simulink model "P2"  (R2014a)
settings: Solver=ode23t  StartTime=0.0  StopTime=0.1  RelTol=1e-3
undefined symbols (not defined in the file): Ts
libraries: powerlib x17, powerlib_extras x5, fl_lib x4, elec_lib x4, nesl_utility x2
settings Model: Creator=HP  LastModifiedBy=HP

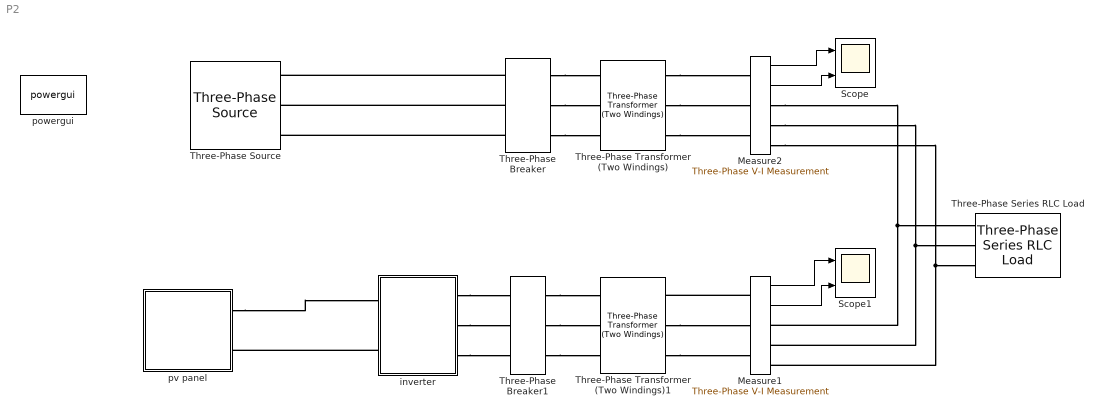
== system P2 ==
  Measure1 : powerlib/Measurements/Three-Phase V-I Measurement  VoltageMeasurement=phase-to-ground  SetLabelV=off  LabelV=V1  Vpu=off  VpuLL=off  CurrentMeasurement=yes  SetLabelI=off  LabelI=I1  Ipu=off  Pbase=1e3  Vbase=380  OutputType=Magnitude  PhasorSimulation=off  PSBequivalent=0
  Measure2 : powerlib/Measurements/Three-Phase V-I Measurement  VoltageMeasurement=phase-to-ground  SetLabelV=off  LabelV=V1  Vpu=off  VpuLL=off  CurrentMeasurement=yes  SetLabelI=off  LabelI=I1  Ipu=off  Pbase=1e3  Vbase=380  OutputType=Magnitude  PhasorSimulation=off  PSBequivalent=0
  Scope : Scope  NumInputPorts=2
      settings: YMin=-5000~-35  YMax=8000~55  SaveName=ScopeData4
  Scope1 : Scope  NumInputPorts=2
      settings: YMin=-2.25~-0.05  YMax=2.75~0.04  SaveName=ScopeData5
  Three-Phase Series RLC Load : powerlib/Elements/Three-Phase Series RLC Load  LConnTagsString=A|B|C  Configuration=Y (grounded)  NominalVoltage=380  NominalFrequency=50  ActivePower=1e3  InductivePower=0  CapacitivePower=0  Measurements=None  LoadType=constant Z
  Three-Phase Transformer (Two Windings) : powerlib/Elements/Three-Phase Transformer (Two Windings)  Winding1Connection=Yg  UNITS=pu  NominalPower=[ 250e6 , 60 ]  Winding1=[ 735e3 , 0.002 , 0.08 ]  Winding2Connection=Yg  Winding2=[ 315e3 , 0.002 , 0.08 ]  SetSaturation=off  Rm=500  Lm=500  Saturation=[ 0,0 ; 0.0024,1.2 ; 1.0,1.52 ]  Hysteresis=off  DataFile='hysteresis'  SetInitialFlux=off  InitialFluxes=[ 0.8 , -0.8 , 0.7 ]  Measurements=None  MoreParameters=off  BreakLoop=off  DataType=off  TransfoNumber=1
  Three-Phase Transformer (Two Windings)1 : powerlib/Elements/Three-Phase Transformer (Two Windings)  Winding1Connection=Yg  UNITS=pu  NominalPower=[ 250e6 , 60 ]  Winding1=[ 735e3 , 0.002 , 0.08 ]  Winding2Connection=Yg  Winding2=[ 315e3 , 0.002 , 0.08 ]  SetSaturation=off  Rm=500  Lm=500  Saturation=[ 0,0 ; 0.0024,1.2 ; 1.0,1.52 ]  Hysteresis=off  DataFile='hysteresis'  SetInitialFlux=off  InitialFluxes=[ 0.8 , -0.8 , 0.7 ]  Measurements=None  MoreParameters=off  BreakLoop=off  DataType=off  TransfoNumber=1
  Three-Phase Breaker : powerlib/Elements/Three-Phase Breaker  InitialState=open  SwitchA=on  SwitchB=on  SwitchC=on  SwitchTimes="[4/60  10/60]"  External=off  BreakerResistance=0.001  SnubberResistance=1e6  SnubberCapacitance=inf  Measurements=None
  Three-Phase Breaker1 : powerlib/Elements/Three-Phase Breaker  InitialState=closed  SwitchA=on  SwitchB=on  SwitchC=on  SwitchTimes="[4/60  10/60]"  External=off  BreakerResistance=0.001  SnubberResistance=1e6  SnubberCapacitance=inf  Measurements=None
  Three-Phase Source : powerlib/Electrical Sources/Three-Phase Source  Voltage=25e3  PhaseAngle=0  Frequency=60  InternalConnection=Yg  SpecifyImpedance=on  Resistance=0.8929  Inductance=16.58e-3  ShortCircuitLevel=100e6  BaseVoltage=25e3  XRratio=7  BusType=swing  Pref=0  Qref=0  Qmin=-inf  Qmax=inf
  inverter : Subsystem
  powergui : powerlib/powergui  Priority=1  SimulationMode=Continuous  SolverType=Tustin  SampleTime=50e-6  frequency=60  SPID=off  DisableSnubberDevices=off  DisableRonSwitches=off  DisableVfSwitches=off  SwTol=0  Interpol=off  DisplayEquations=off  Ts=0  methode=off  frequencyindice=0  Pbase=100e6  ErrMax=1e-4  Iterations=50  UnitsV=kV  UnitsW=MW  FunctionMessages=off  echomessages=off  HookPort=off  EnableUseOfTLC=off  x0status=blocks  RestoreLinks=warning  ResistiveCurrentMeasurement=off  Frange=[0:2:500]  Ylog=off  Xlog=on  ShowGrid=off  save=off  variable=ZData  structure=0  ZoomFFT=off  StartTime=0.0  cycles=1  DisplayStyle=1  fundamental=60  FreqAxis=off  MaxFrequency=1000  frequencyindicesteady=1  RmsSteady=1  display=off
  pv panel : Subsystem
  wires:
  Measure2/1 -> Scope/1
  Measure2/2 -> Scope/2
  Measure1/2 -> Scope1/2
  Measure1/1 -> Scope1/1
  connections:
  Measure2/RConn3 -- Measure1/RConn3 -- Three-Phase Series RLC Load/LConn3
  Measure2/RConn2 -- Measure1/RConn2 -- Three-Phase Series RLC Load/LConn2
  Measure2/RConn1 -- Measure1/RConn1 -- Three-Phase Series RLC Load/LConn1
  Three-Phase Breaker/LConn3 -- Three-Phase Source/RConn3
  Three-Phase Breaker/LConn2 -- Three-Phase Source/RConn2
  Three-Phase Breaker/LConn1 -- Three-Phase Source/RConn1
  inverter/RConn1 -- Three-Phase Breaker1/LConn1
  inverter/RConn2 -- Three-Phase Breaker1/LConn2
  inverter/RConn3 -- Three-Phase Breaker1/LConn3
  Three-Phase Breaker1/RConn1 -- Three-Phase Transformer (Two Windings)1/LConn1
  Three-Phase Breaker1/RConn2 -- Three-Phase Transformer (Two Windings)1/LConn2
  Three-Phase Breaker1/RConn3 -- Three-Phase Transformer (Two Windings)1/LConn3
  Measure1/LConn1 -- Three-Phase Transformer (Two Windings)1/RConn1
  Three-Phase Transformer (Two Windings)1/RConn2 -- Measure1/LConn2
  Three-Phase Transformer (Two Windings)1/RConn3 -- Measure1/LConn3
  pv panel/RConn1 -- inverter/LConn1
  inverter/LConn2 -- pv panel/RConn2
  Three-Phase Breaker/RConn1 -- Three-Phase Transformer (Two Windings)/LConn1
  Three-Phase Breaker/RConn2 -- Three-Phase Transformer (Two Windings)/LConn2
  Three-Phase Breaker/RConn3 -- Three-Phase Transformer (Two Windings)/LConn3
  Three-Phase Transformer (Two Windings)/RConn1 -- Measure2/LConn1
  Three-Phase Transformer (Two Windings)/RConn2 -- Measure2/LConn2
  Three-Phase Transformer (Two Windings)/RConn3 -- Measure2/LConn3

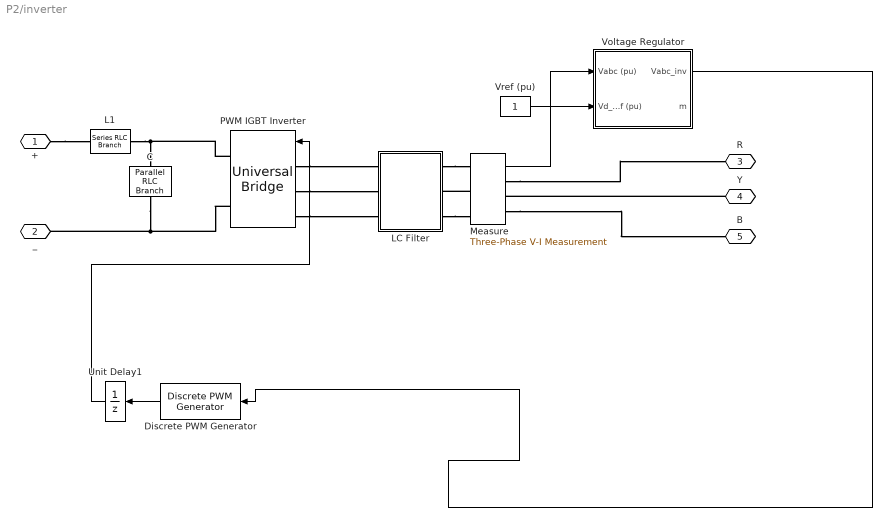
== system P2/inverter ==
  C : powerlib/Elements/Parallel RLC Branch  LConnTagsString=a  RConnTagsString=__new0  BranchType=RLC  Resistance=inf  Inductance=inf  SetiL0=off  InitialCurrent=0  Capacitance=5000e-06  Setx0=off  InitialVoltage=0  Measurements=None
  Discrete PWM Generator : powerlib_extras/Discrete  Control Blocks/Discrete PWM Generator  GeneratorMode="3-arm  bridge (6 pulses)"  Fc=2000  Ts=Ts  Internal=off  mIndex=0.4  Freq=60  Phase=0
  L1 : powerlib/Elements/Series RLC Branch  LConnTagsString=__new0  RConnTagsString=__new0  BranchType=L  Resistance=1.0  Inductance=200e-6  SetiL0=off  InitialCurrent=0  Capacitance=1.0  Setx0=off  InitialVoltage=0  Measurements=None
  LC Filter : Subsystem
  Measure : powerlib/Measurements/Three-Phase V-I Measurement  VoltageMeasurement=phase-to-ground  SetLabelV=off  LabelV=V1  Vpu=on  VpuLL=off  CurrentMeasurement=no  SetLabelI=off  LabelI=I1  Ipu=off  Pbase=1e3  Vbase=380  OutputType=Magnitude  PhasorSimulation=off  PSBequivalent=0
  PWM IGBT Inverter : powerlib/Power Electronics/Universal Bridge  Arms=3  SnubberResistance=5000  SnubberCapacitance=inf  Device=IGBT / Diodes  Ron=1e-3  Lon=0  ForwardVoltages="[  0.0  0.0  ]"  ForwardVoltage=.8  GTOparameters=[ 1e-6 ,1e-6 ]  IGBTparameters=[ 1e-6 , 2e-6 ]  Measurements=Device currents  Measurements_2=None  converterType=Rectifier
  Unit Delay1 : UnitDelay  SampleTime=Ts
  Voltage Regulator : Subsystem  mask(Voltage Regulator){Kp=0.4, Ki=500, Ts=Ts}
      mask prompts: Kp "Proportional gain  Kp:"; Ki "Integral gain Ki:"; Ts "Sample time (s) :"
  "Vref (pu) " : Constant
  + : PMIOPort  Port=1  Side=Left
  _ : PMIOPort  Port=2  Side=Left
  R : PMIOPort  Port=3  Side=Right
  Y : PMIOPort  Port=4  Side=Right
  B : PMIOPort  Port=5  Side=Right
  wires:
  "Vref (pu) "/1 -> Voltage Regulator/2(Vd_ref (pu))
  Discrete PWM Generator/1 -> Unit Delay1/1
  Voltage Regulator/1(Vabc_inv) -> Discrete PWM Generator/1
  Unit Delay1/1 -> PWM IGBT Inverter/1
  Measure/1 -> Voltage Regulator/1(Vabc (pu))
  connections:
  PWM IGBT Inverter/RConn2 -- C/RConn1 -- _/RConn1
  PWM IGBT Inverter/RConn1 -- L1/RConn1 -- C/LConn1
  PWM IGBT Inverter/LConn2 -- LC Filter/LConn2
  PWM IGBT Inverter/LConn1 -- LC Filter/LConn1
  Y/RConn1 -- Measure/RConn2
  Measure/RConn1 -- R/RConn1
  Measure/LConn2 -- LC Filter/RConn2
  Measure/RConn3 -- B/RConn1
  PWM IGBT Inverter/LConn3 -- LC Filter/LConn3
  LC Filter/RConn1 -- Measure/LConn1
  LC Filter/RConn3 -- Measure/LConn3
  +/RConn1 -- L1/LConn1

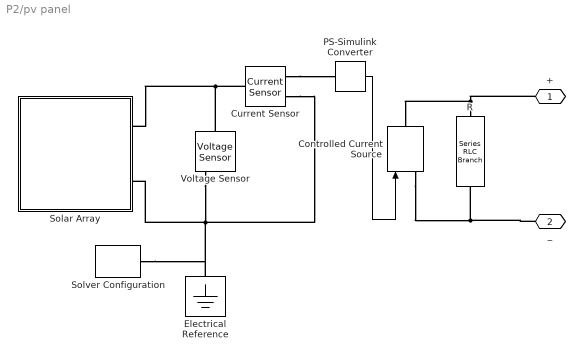
== system P2/pv panel ==
  " R " : powerlib/Elements/Series RLC Branch  LConnTagsString=__new0  RConnTagsString=__new0  BranchType=R  Resistance=10  Inductance=1e-3  SetiL0=off  InitialCurrent=0  Capacitance=1e-6  Setx0=off  InitialVoltage=0  Measurements=None
  Controlled Current Source : powerlib/Electrical Sources/Controlled Current Source  Initialize=on  Source_Type=AC  Amplitude=0  Phase=0  Frequency=0  Measurements=None
  Current Sensor : fl_lib/Electrical/Electrical Sensors/Current Sensor
  Electrical Reference : fl_lib/Electrical/Electrical Elements/Electrical Reference
  PS-Simulink Converter : nesl_utility/PS-Simulink Converter  PhysicalDomain=network_engine_domain  SubClassName=ps_output  LeftPortType=input  RightPortType=output  PseudoPeriodic=off  Frequencies=[]  Unit=1  AffineConversion=off
  Solar Array : Subsystem
  Solver Configuration : nesl_utility/Solver Configuration  PhysicalDomain=network_engine_domain  SubClassName=solver  LeftPortType=input  RightPortType=generic  Accelerate=off  Tones=[]  Harmonics=[]  SimulateNoise=off  Profile=off  UseLocalSampling=off  EnableSwitchedLinearOptims=on  FrequencyDomain=off  UseCCode=off  RelTol=0.001  AbsTol=1e-06  MinStep=1e-09  ToWorkspace=off  DoDC=off  ResidualTolerance=1e-9  UseLocalSolver=off  LocalSolverChoice=NE_BACKWARD_EULER_ADVANCER  LocalSolverSampleTime=.001  DoFixedCost=off  MaxNonlinIter=3  MaxModeIter=2  LinearAlgebra=Sparse  DelaysMemoryBudget=1024  AutomaticFiltering=on  FilteringTimeConstant=0.001
  Voltage Sensor : fl_lib/Electrical/Electrical Sensors/Voltage Sensor
  + : PMIOPort  Port=1  Side=Right
  _ : PMIOPort  Port=2  Side=Right
  wires:
  PS-Simulink Converter/1 -> Controlled Current Source/1
  connections:
  Controlled Current Source/LConn1 -- " R "/RConn1 -- _/RConn1
  " R "/LConn1 -- +/RConn1 -- Controlled Current Source/RConn1
  Current Sensor/RConn1 -- PS-Simulink Converter/LConn1
  Voltage Sensor/RConn2 -- Solar Array/RConn2 -- Solver Configuration/RConn1 -- Electrical Reference/LConn1 -- Current Sensor/RConn2
  Current Sensor/LConn1 -- Voltage Sensor/LConn1 -- Solar Array/RConn1

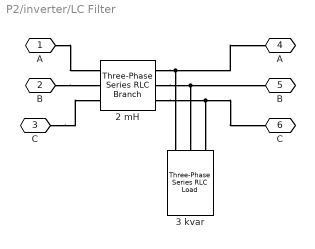
== system P2/inverter/LC Filter ==
  "2 mH " : powerlib/Elements/Three-Phase Series RLC Branch  LConnTagsString=A|B|C  RConnTagsString=A|B|C  BranchType=L  Resistance=1.0  Inductance=2e-3  Capacitance=1.0  Measurements=None
  3 kvar : powerlib/Elements/Three-Phase Series RLC Load  LConnTagsString=A|B|C  Configuration=Y (grounded)  NominalVoltage=380  NominalFrequency=50  ActivePower=0  InductivePower=0  CapacitivePower=3e3  Measurements=None  LoadType=constant Z
  A : PMIOPort  Port=1  Side=Left
  B : PMIOPort  Port=2  Side=Left
  C : PMIOPort  Port=3  Side=Left
  "A " : PMIOPort  Port=4  Side=Right
  "B " : PMIOPort  Port=5  Side=Right
  "C " : PMIOPort  Port=6  Side=Right
  connections:
  B/RConn1 -- "2 mH "/LConn2
  A/RConn1 -- "2 mH "/LConn1
  C/RConn1 -- "2 mH "/LConn3
  "2 mH "/RConn1 -- "A "/RConn1 -- 3 kvar/LConn1
  "2 mH "/RConn2 -- "B "/RConn1 -- 3 kvar/LConn2
  "2 mH "/RConn3 -- "C "/RConn1 -- 3 kvar/LConn3

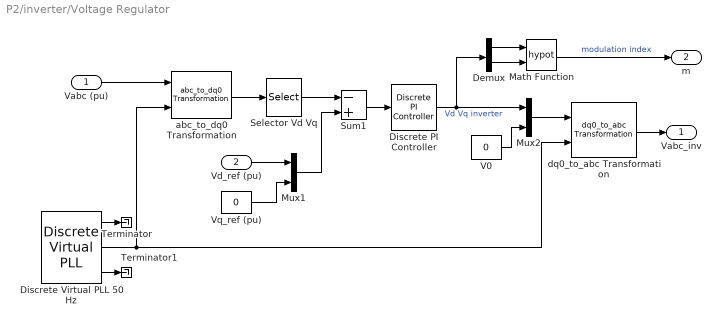
== system P2/inverter/Voltage Regulator ==
  Vabc (pu) : Inport
  Vd_ref (pu) : Inport  Port=2
  Demux : Demux  Outputs=2
  Discrete PI Controller : powerlib_extras/Discrete  Control Blocks/Discrete PI Controller  Kp=Kp  Ki=Ki  Par_Limits=[1 -1]  Init=0  Ts=Ts
  Discrete Virtual PLL 50 Hz : powerlib_extras/Discrete  Control Blocks/Discrete Virtual PLL  Freq=50  Phase=0  Ts=Ts
  Math Function : Math  Operator=hypot  SaturateOnIntegerOverflow=on
  Mux1 : Mux  Inputs=2
  Mux2 : Mux  Inputs=2
  Selector Vd Vq : Selector  InputPortWidth=3  Indices=[1 2]
  Sum1 : Sum  Inputs=-+  SaturateOnIntegerOverflow=on  InputSameDT=on  OutDataTypeStr=Inherit: Same as first input
  Terminator : Terminator
  Terminator1 : Terminator
  V0 : Constant  Value=0
  Vq_ref (pu) : Constant  Value=0
  abc_to_dq0 Transformation : powerlib_extras/Measurements/abc_to_dq0 Transformation
  dq0_to_abc Transformation : powerlib_extras/Measurements/dq0_to_abc Transformation
  Vabc_inv : Outport
  m : Outport  Port=2
  wires:
  abc_to_dq0 Transformation/1 -> Selector Vd Vq/1
  Vabc (pu)/1 -> abc_to_dq0 Transformation/1
  Selector Vd Vq/1 -> Sum1/1
  Sum1/1 -> Discrete PI Controller/1
  Mux2/1 -> dq0_to_abc Transformation/1
  V0/1 -> Mux2/2
  dq0_to_abc Transformation/1 -> Vabc_inv/1
  Discrete Virtual PLL 50 Hz/2 -> abc_to_dq0 Transformation/2, dq0_to_abc Transformation/2
  Vd_ref (pu)/1 -> Mux1/1
  Vq_ref (pu)/1 -> Mux1/2
  Mux1/1 -> Sum1/2
  Discrete Virtual PLL 50 Hz/1 -> Terminator/1
  Discrete Virtual PLL 50 Hz/3 -> Terminator1/1
  Discrete PI Controller/1 -> Demux/1, Mux2/1  "Vd Vq inverter"
  Demux/1 -> Math Function/1
  Demux/2 -> Math Function/2
  Math Function/1 -> m/1  "modulation index"

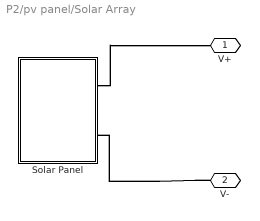
== system P2/pv panel/Solar Array ==
  Solar Panel : Subsystem
  V+ : PMIOPort  Port=1  Side=Right
  V- : PMIOPort  Port=2  Side=Right
  connections:
  Solar Panel/RConn1 -- V+/RConn1
  V-/RConn1 -- Solar Panel/RConn2

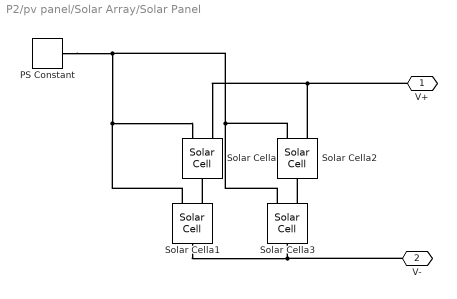
== system P2/pv panel/Solar Array/Solar Panel ==
  PS Constant : fl_lib/Physical Signals/Sources/PS Constant  constant=687
  Solar Cella{,1..3} (4 alike) : elec_lib/Sources/Solar Cell  prm=1  Isc=8.20 A  Voc=3.655 V  Is=1e-6 A  Is2=0 A  Iph=7.34 A  Ir0=1000 W/m^2  ec=1.6  N2=2  Rs=5.1e-3 Ohm  Rp=Inf Ohm  N_series=10  TIPH1=0.65e-3 1/K  EG=1.12 eV  TXIS1=3  TXIS2=3  TRS1=0  TRP1=0  Tmeas=25 C  TFIXED=25 C  thermal_mass=100 J/K  initial_temperature=25 C
  V+ : PMIOPort  Port=1  Side=Right
  V- : PMIOPort  Port=2  Side=Right
  connections:
  PS Constant/RConn1 -- Solar Cella2/LConn1 -- Solar Cella3/LConn1 -- Solar Cella1/LConn1 -- Solar Cella/LConn1
  V+/RConn1 -- Solar Cella2/LConn2 -- Solar Cella/LConn2
  Solar Cella1/LConn2 -- Solar Cella/RConn1
  Solar Cella3/LConn2 -- Solar Cella2/RConn1
  Solar Cella1/RConn1 -- V-/RConn1 -- Solar Cella3/RConn1
